simulink library "DoorHndReq"  (R2022a)
settings: Solver=VariableStepAuto  StartTime=0.0  StopTime=10.0  RelTol=1e-3
settings Model: Creator=DELL  LastModifiedBy=DELL

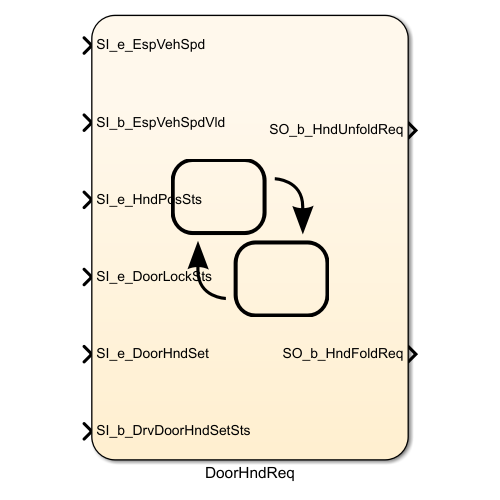
[thumbnail: Simulink's stored preview of the top-level diagram]
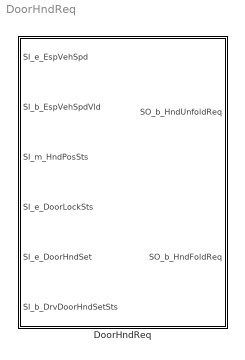
== system DoorHndReq ==
  DoorHndReq : Stateflow chart  TreatAsAtomicUnit=on

== stateflow chart DoorHndReq/DoorHndReq ==
  state AntiPlay [parallel]
    settings: executionOrder=3
    state Count
      (default) -> (junction 654)
      Count -> (junction 654) [order 1]
      (junction 654) -> (junction 655) [order 1] : [hasChangedTo(SI_m_HndPosSts, Hnd_Fold) || ...
          | hasChangedTo(SI_m_HndPosSts, Hnd_Unfold)]
      (junction 654) -> (junction 656) [order 2]
      (junction 655) -> (junction 662) : {SL_e_antiPlayCount ++}
      (junction 662) -> (junction 656)
      (junction 656) -> (junction 658)
    state TrigAndClean
      en:
      SL_b_antiPlayFlg = 1;
      SL_e_antiPlayCount = 0;
    state Clean
      en:
      SL_e_antiPlayCount = 0;
    (default) -> Count
    Count -> TrigAndClean [order 1] : [before(3000, tick) &&...
        | SL_e_antiPlayCount >= 10]
    TrigAndClean -> Count : after(18000, tick)
        | {SL_b_antiPlayFlg = 0;}
    Count -> Clean [order 2] : [after(3000, tick)]
    Clean -> Count
  state Unfold [parallel]
    settings: executionOrder=1
    state Idle
      SO_b_HndUnfoldReq = 0;
    state NormalUnfoldReq
      en:
      SO_b_HndUnfoldReq = 1;
      on at(5, tick):
      SO_b_HndUnfoldReq = 0;
    state ExhibUnfoldReq
      en:
      SO_b_HndUnfoldReq = 1;
    state WashUnfoldReq
      en:
      SO_b_HndUnfoldReq = 1;
    (default) -> Unfold.Idle
    Unfold.Idle -> NormalUnfoldReq [order 1] : [((SI_e_EspVehSpd <= 20 && SI_b_EspVehSpdVld == 0) || ...
        | SI_b_EspVehSpdVld == 1) && ...
        | (SI_b_DoorAjar == 1 || SI_e_DoorLockSts == 1) && ...
        | SI_m_HndPosSts != Hnd_Unfold]
    NormalUnfoldReq -> Unfold.Idle : [(SI_e_EspVehSpd > 20 && SI_b_EspVehSpdVld == 0) || ...
        | (SI_b_DoorAjar != 1 && SI_e_DoorLockSts != 1) || ...
        | SI_m_HndPosSts == Hnd_Unfold]
    Unfold.Idle -> ExhibUnfoldReq [order 2] : [hasChangedTo(SI_e_DoorHndSet, 4) && ...
        | SI_m_HndPosSts != Hnd_Unfold]
    ExhibUnfoldReq -> Unfold.Idle : after(5, tick)
    Unfold.Idle -> WashUnfoldReq [order 3] : [hasChangedTo(SI_e_DoorHndSet, 3) && ...
        | SI_m_HndPosSts != Hnd_Unfold]
    WashUnfoldReq -> Unfold.Idle : after(5, tick)
  state Fold [parallel]
    settings: executionOrder=2
    state Idle
      SO_b_HndFoldReq = 0;
    state FoldReq
      en:
      SO_b_HndFoldReq = 1;
      on at(5, tick):
      SO_b_HndFoldReq = 0;
    (default) -> Fold.Idle
    Fold.Idle -> FoldReq : [(SI_e_EspVehSpd > 20 && SI_b_EspVehSpdVld == 0) && ...
        | SI_e_DoorLockSts == 0 && ...
        | SL_b_antiPlayFlg == 0 && ...
        | SI_m_HndPosSts != Hnd_Fold && ...
        | SI_b_DrvDoorHndSetSts == 0]
    FoldReq -> Fold.Idle : [((SI_e_EspVehSpd <= 20 && SI_b_EspVehSpdVld == 0) || ...
        | SI_b_EspVehSpdVld == 1) || ...
        | SI_e_DoorLockSts != 0 || ...
        | SL_b_antiPlayFlg == 1 || ...
        | SI_m_HndPosSts == Hnd_Fold || ...
        | SI_b_DrvDoorHndSetSts == 1]
  data: SI_e_EspVehSpd input uint8; SI_b_EspVehSpdVld input boolean; SO_b_HndUnfoldReq output boolean; SL_e_antiPlayCount local uint8 =0; SI_m_HndPosSts input Enum: HndPos_Sts_E; SI_e_DoorLockSts input uint8; SI_e_DoorHndSet input uint8; SO_b_HndFoldReq output boolean; SI_b_DrvDoorHndSetSts input boolean =0; SL_b_antiPlayFlg local uint8 =0
